simulink model "flight_sim"  (R2022b)
settings: Solver=ode45  StartTime=0.0  StopTime=304.15  RelTol=1e-3
values from neighbouring files (symbols this model uses):
  g = 9.81    [parameters.m]
  gam_0 = pi/2    (= 1.57079632679)    [parameters.m]
  gam_in = 0.10    (= 0.1)    [parameters.m]
  h_0 = 6    [parameters.m]
  m_dot = 132    [parameters.m]
  m_zfw = m_pay + m_dry    (= 6360.7)    [parameters.m]
  R_E = 6371e3    (= 6371000)    [parameters.m]
  t_turn = 30.0    (= 30)    [parameters.m]
  v_0 = 0.01    [parameters.m]
  x_0 = 0    [parameters.m]
undefined symbols (not defined in the file or in its folder): Earth, WGS84
libraries: aerolibfltsims x1, aerolibanim x1, aerolibtransform2 x1, slpidlib x1, simulink x1
settings Model: Creator=Utilizador  LastModifiedBy=alexa
settings ModelReferenceCC: EnableRefExpFcnMdlSchedulingChecks=on

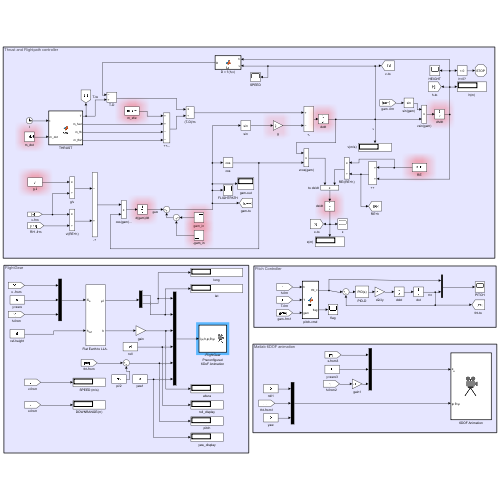
[thumbnail: Simulink's stored preview of the top-level diagram]
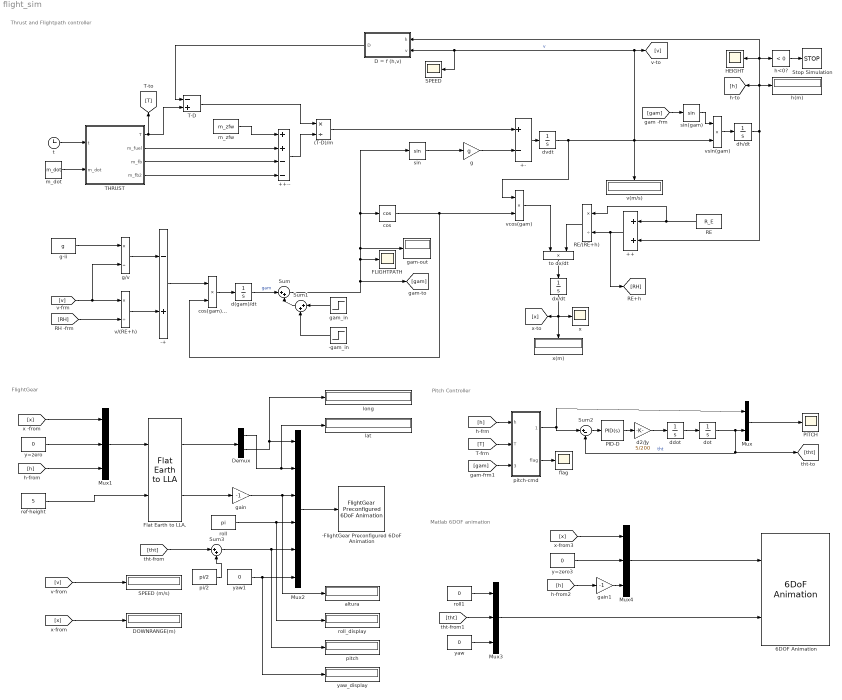
== system flight_sim ==
  note: Matlab 6DOF animation
  note: FlightGear
  note: Thrust and Flightpath controller
  note: Pitch Controller
  (T-D)/m : Product  Inputs=*/
  ++ : Sum
  ++-- : Sum  Inputs=++--
  +- : Sum  Inputs=+-
  -+ : Sum  Inputs=-+
  -FlightGear Preconfigured 6DoF Animation : aerolibfltsims/FlightGear Preconfigured 6DoF Animation  xFlightGearVersion=v2019.1  DestinationIpAddress=127.0.0.1  DestinationPort=5502  SampleTime=1/30  packetVersion=24
  -gam_in : Step  Time=t_turn+1  Before=-gam_in  After=-gam_in  SampleTime=0
  6DOF Animation : aerolibanim/6DoF Animation  u1=[0 4000 -2000 2000 -5000 -3000]  u2=0.1  u3=1.0  u4=[4000 0 -5000]  u5=Fixed position  u6=[2000 500 -3150]  u7=10  u8=on
  D = f (h,v) : MATLAB Function  TreatAsAtomicUnit=on
  DOWNRANGE(m) : Display
  Demux : Demux  Outputs=2
  FLIGHTPATH : Scope
  "Flat Earth to LLA. " : aerolibtransform2/Flat Earth to LLA  units=Metric (MKS)  ptype=Earth (WGS84)  F=1/298.257223563  R=6378137  refPosPort=off  LL0=[28.48573 -80.54295]  psi=0
  HEIGHT : Scope
  Mux : Mux  Inputs=2
  Mux1 : Mux  Inputs=3
  Mux2 : Mux  Inputs=6
  Mux3 : Mux  Inputs=3
  Mux4 : Mux  Inputs=3
  PID-D : slpidlib/PID Controller  Controller=PID  Form=Parallel  TimeDomain=Continuous-time  UseExternalTs=off  SampleTime=-1  IntegratorMethod=Forward Euler  FilterMethod=Forward Euler  ControllerParametersSource=internal  P=0  I=0  UseKiTs=off  D=200/5  N=100  UseFilter=on  TunerSelectOption=Transfer Function Based (PID Tuner App)  InitialConditionSource=internal  InitialConditionForIntegrator=0  InitialConditionForFilter=0  DifferentiatorICPrevScaledInput=0  ExternalReset=none  TrackingMode=off  Kt=1  LimitOutput=off  SatLimitsSource=internal  UpperSaturationLimit=inf  LowerSaturationLimit=-inf  LinearizeAsGain=on  AntiWindupMode=none  Kb=1  LimitIntegrator=off  UpperIntegratorSaturationLimit=inf  LowerIntegratorSaturationLimit=-inf  POutMin=[]  POutMax=[]  IOutMin=[]  IOutMax=[]  DOutMin=[]  DOutMax=[]  NOutMin=[]  NOutMax=[]  SumOutMin=[]  SumOutMax=[]  SaturationOutMin=[]  SaturationOutMax=[]  PParamMin=[]  PParamMax=[]  IParamMin=[]  IParamMax=[]  DParamMin=[]  DParamMax=[]  NParamMin=[]  NParamMax=[]  KbParamMin=[]  KbParamMax=[]  KtParamMin=[]  KtParamMax=[]  KbOutMin=[]  KbOutMax=[]  KtOutMin=[]  KtOutMax=[]  IntegratorOutMin=[]  IntegratorOutMax=[]  FilterOutMin=[]  FilterOutMax=[]  SumI1OutMin=[]  SumI1OutMax=[]  SumI2OutMin=[]  SumI2OutMax=[]  SumI3OutMin=[]  SumI3OutMax=[]  SumI4OutMin=[]  SumI4OutMax=[]  SumDOutMin=[]  SumDOutMax=[]  DifferentiatorOutMin=[]  DifferentiatorOutMax=[]  FilterDiffOutCoefMin=[]  FilterDiffOutCoefMax=[]  ReciprocalOutMin=[]  ReciprocalOutMax=[]  SumDenOutMin=[]  SumDenOutMax=[]  SumNumOutMin=[]  SumNumOutMax=[]  DivideOutMin=[]  DivideOutMax=[]  UdiffTsProdOutMin=[]  UdiffTsProdOutMax=[]  NTsProdOutMin=[]  NTsProdOutMax=[]  UintegralTsProdOutMin=[]  UintegralTsProdOutMax=[]  UngainTsProdOutMin=[]  UngainTsProdOutMax=[]  ClampingZeroOutDataTypeStr=Inherit: Inherit via back propagation  ClampingZeroOutMin=[]  ClampingZeroOutMax=[]  FilterDenConstantOutDataTypeStr=Inherit: Inherit via back propagation  FilterDenConstantOutMin=[]  FilterDenConstantOutMax=[]  PCopyOutDataTypeStr=Inherit: Inherit via back propagation  PCopyOutMin=[]  PCopyOutMax=[]  NCopyOutDataTypeStr=Inherit: Inherit via back propagation  NCopyOutMin=[]  NCopyOutMax=[]  IntegratorContinuousStateAttributes=''  IntegratorStateMustResolveToSignalObject=off  IntegratorRTWStateStorageClass=Auto  FilterContinuousStateAttributes=''  FilterStateMustResolveToSignalObject=off  FilterRTWStateStorageClass=Auto  ParallelPVariant=InternalParameters  IdealPVariant=Disabled  IVariant=InternalParameters  DVariant=InternalParameters  IntegratorVariant=Continuous  SatVariant=Disabled  AWVariant=Passthrough  PCopyVariant=Disabled  TRVariant=Disabled  FdbkBlocksVariant=Forward  IdealPFdbkVariant=Disabled  SatFdbkVariant=Disabled  DerivativeFilterVariant=ContFilter  NVariant=InternalParameters  NCopyVariant=Disabled  FilterICVariant=InternalICsFilter  IntegratorICVariant=InternalICs  ExternalResetVariant=Disabled  TRSumVariant=Passthrough  SumFdbkVariant=Disabled  SumVariant=Sum_PID  TsampFilterVariant=InternalTs  TsampNgainVariant=Passthrough  TsampIntegralVariant=Passthrough  ExternalSaturationOutDataTypeStr=Inherit: Same as second input
  PITCH : Scope
  RE : Constant  Value=R_E
  RE/(RE+h) : Product  Inputs=*/
  SPEED : Scope
  SPEED (m/s) : Display
  Stop Simulation : Stop
  Sum : Sum  Inputs=|++
  Sum1 : Sum  Inputs=|++
  Sum2 : Sum  Inputs=|+-
  Sum3 : Sum  Inputs=|++
  T-D : Sum  Inputs=-+
  THRUST : MATLAB Function  TreatAsAtomicUnit=on
  altura : Display
  cos : Trigonometry  Operator=cos
  cos(gam)... : Product
  d(gam)/dt : Integrator  InitialCondition=gam_0
  d2/Jy : Gain  Gain=5/200
  ddot : Integrator
  dh/dt : Integrator  InitialCondition=h_0
  dot : Integrator  InitialCondition=pi/2
  dvdt : Integrator  InitialCondition=v_0
  dx/dt : Integrator  InitialCondition=x_0
  flag : Scope
  g : Gain  Gain=g
  g-ii : Constant  Value=g
  g/v : Product  Inputs=*/
  gain : Gain  Gain=-1
  gain1 : Gain  Gain=-1
  gam-out : Display
  gam_in : Step  Time=t_turn  Before=gam_in  After=0  SampleTime=0
  h(m) : Display
  h<0? : simulink/Logic and Bit Operations/Compare To Zero  relop=<  OutDataTypeStr=boolean
  lat : Display
  long : Display
  m_dot : Constant  Value=m_dot
  m_zfw : Constant  Value=m_zfw
  pi/2 : Constant  Value=pi/2
  pitch : Display
  pitch-cmd : MATLAB Function  TreatAsAtomicUnit=on
  ref-height : Constant  Value=5
  roll : Constant  Value=pi
  roll1 : Constant  Value=0
  roll_display : Display
  sin : Trigonometry
  sin(gam) : Trigonometry
  t : Clock
  to dx/dt : Product
  v(m/s) : Display
  v/(RE+h) : Product  Inputs=*/
  vcos(gam) : Product
  vsin(gam) : Product
  x : Scope
  x(m) : Display
  y=zero : Constant  Value=0
  y=zero3 : Constant  Value=0
  yaw : Constant  Value=0
  yaw1 : Constant  Value=0
  yaw_display : Display
  wires:
  t/1 -> THRUST/1(t)
  m_dot/1 -> THRUST/2(m_dot)
  THRUST/1(T) -> T-D/2, [T]
  m_zfw/1 -> ++--/1
  THRUST/3(m_fb) -> ++--/3
  THRUST/4(m_fb2) -> ++--/4
  THRUST/2(m_fuel) -> ++--/2
  T-D/1 -> (T-D)/m/1
  ++--/1 -> (T-D)/m/2
  (T-D)/m/1 -> +-/1
  g/1 -> +-/2
  sin/1 -> g/1
  +-/1 -> dvdt/1
  dvdt/1 -> v(m/s)/1, vsin(gam)/2, D = f (h,v)/2(v), SPEED/1, [v], vcos(gam)/1  "v"
  dh/dt/1 -> ++/2, h(m)/1, h<0?/1, D = f (h,v)/1(h), HEIGHT/1, [h]
  h<0?/1 -> Stop Simulation/1
  D = f (h,v)/1(D) -> T-D/1
  ++/1 -> [RH], RE/(RE+h)/2
  RE/1 -> ++/1, RE/(RE+h)/1
  RE/(RE+h)/1 -> to dx/dt/2
  to dx/dt/1 -> dx/dt/1
  g-ii/1 -> g/v/1
  [v] -> g/v/2, v/(RE+h)/1
  [RH] -> v/(RE+h)/2
  g/v/1 -> -+/1
  v/(RE+h)/1 -> -+/2
  -+/1 -> cos(gam).../1
  cos(gam).../1 -> d(gam)/dt/1
  d(gam)/dt/1 -> Sum/1  "gam"
  Sum/1 -> [gam], FLIGHTPATH/1, cos/1, sin/1, gam-out/1
  vcos(gam)/1 -> to dx/dt/1
  sin(gam)/1 -> vsin(gam)/1
  [gam] -> sin(gam)/1
  gam_in/1 -> Sum1/1
  -gam_in/1 -> Sum1/2
  Sum1/1 -> Sum/2
  cos/1 -> vcos(gam)/2, cos(gam).../2
  [h] -> pitch-cmd/1(h)
  [T] -> pitch-cmd/2(T)
  [gam] -> pitch-cmd/3(gam)
  pitch-cmd/2(flag) -> flag/1
  pitch-cmd/1(tht_c) -> Mux/1, Sum2/1
  Sum2/1 -> PID-D/1
  PID-D/1 -> d2/Jy/1
  d2/Jy/1 -> ddot/1
  ddot/1 -> dot/1
  dot/1 -> Sum2/2, [tht], Mux/2  "tht"
  Mux/1 -> PITCH/1
  vsin(gam)/1 -> dh/dt/1
  dx/dt/1 -> [x], x/1, x(m)/1
  [x] -> Mux1/1
  [h] -> Mux1/3
  y=zero/1 -> Mux1/2
  Mux1/1 -> "Flat Earth to LLA. "/1
  ref-height/1 -> "Flat Earth to LLA. "/2
  "Flat Earth to LLA. "/1 -> Demux/1
  "Flat Earth to LLA. "/2 -> gain/1
  gain/1 -> altura/1, Mux2/3
  roll/1 -> roll_display/1, Mux2/4
  Mux2/1 -> -FlightGear Preconfigured 6DoF Animation/1
  [v] -> SPEED (m/s)/1
  [x] -> DOWNRANGE(m)/1
  roll1/1 -> Mux3/1
  yaw/1 -> Mux3/3
  [x] -> Mux4/1
  y=zero3/1 -> Mux4/2
  gain1/1 -> Mux4/3
  [h] -> gain1/1
  Mux4/1 -> 6DOF Animation/1
  Mux3/1 -> 6DOF Animation/2
  [tht] -> Mux3/2
  yaw1/1 -> yaw_display/1, Mux2/6
  Demux/2 -> long/1, Mux2/1
  Demux/1 -> lat/1, Mux2/2
  [tht] -> Sum3/1
  Sum3/1 -> pitch/1, Mux2/5
  pi/2/1 -> Sum3/2

== matlab function flight_sim/pitch-cmd ==
  settings: updateMethod=DISCRETE
  data: h input; tht_c output; T input; gam input; flag output
function [tht_c, flag] = fcn(h,T,gam)

persistent f

if isempty(f)
	f = 0;
end
if T<=0
	t_c = gam+pi;
	if t_c>pi
		t_c = pi;
	end
	f = 1;
elseif T<=0 && h<1000
	t_c = pi/2;
else
	t_c = gam;
end
flag = f;
tht_c = t_c;

== matlab function flight_sim/THRUST ==
  settings: updateMethod=DISCRETE
  data: t input; T output; m_fuel output; m_fb output; m_fb2 output; m_dot input
function [T, m_fuel, m_fb, m_fb2] = fcn(t,m_dot)
%#codegen

persistent mfb
persistent mfb2

if isempty(mfb)
	mfb = 0;
end
if isempty(mfb2)
	mfb2 = 0;
end

mfuel = 21491.26;

if mfb <= 0.65*mfuel
	THR = 346961.2;
	mfb = t*m_dot;
else
	THR = 0;
end

if (125<t) && (t<295)
	THR = -110000;
	mfb2 = (t-125)*(m_dot/3);
end

T = THR;
m_fb = mfb;
m_fb2 = mfb2;
m_fuel = mfuel;

== matlab function flight_sim/D = f (h,v) ==
  data: h input; D output; v input
function D = fcn(h,v)

CD = 0.075;

Di = 1.5;

A = pi*Di^2/4;

%density ISA model
if h<= 11000
	T = 15.04 - 0.00649*h;
	p = 101.29*((T+273.1)/288.88)^5.258;
elseif (11000<h) && (h<=25000)
	T = -56.46;
	p = 22.65*exp(1.73-0.000157*h);

else
	T = -131.21 + 0.00299*h;
	p = 2.488*((T+273.1)/216.6)^-11.388;
end

rho = p/(0.2869*(T+273.1));

%drag force D
Drag = 0.5*rho*v^2*A*CD;

D = Drag;
